simulink model "Task19"  (R2022b)
settings: Solver=VariableStepAuto  StartTime=0.0  StopTime=10.0  RelTol=1e-3
libraries: simulink x1
settings Model: Creator=LOQ  LastModifiedBy=LOQ
settings OptimizationCC: ReuseModelBlockBuffer=on
settings RTWCC: GPUComputeCapability=5.0
settings ConfigComp: CovBoundaryAbsTol=1.0e-5

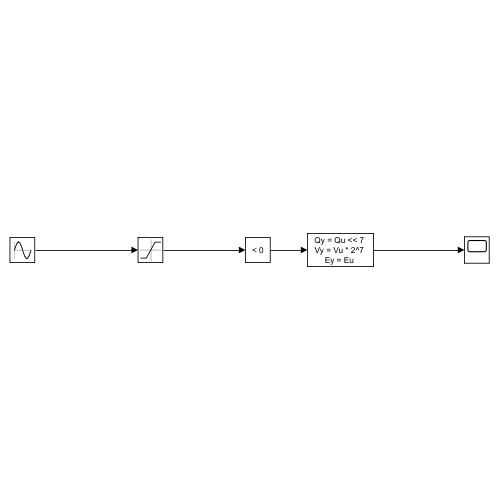
[thumbnail: Simulink's stored preview of the top-level diagram]
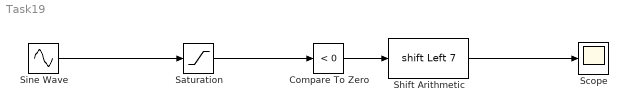
== system Task19 ==
  Compare To Zero : simulink/Logic and Bit Operations/Compare To Zero  relop=<  OutDataTypeStr=uint8
  Saturation : Saturate  UpperLimit=5  LowerLimit=-5
  Scope : Scope
  Shift Arithmetic : ArithShift  BitShiftNumber=7  BitShiftDirection=Left
  Sine Wave : Sin  SampleTime=0
  wires:
  Saturation/1 -> Compare To Zero/1
  Sine Wave/1 -> Saturation/1
  Compare To Zero/1 -> Shift Arithmetic/1
  Shift Arithmetic/1 -> Scope/1
